simulink subsystem "PID_mask"  (R2022b)
settings: Solver=VariableStepAuto  StartTime=0.0  StopTime=10.0  RelTol=1e-3
model mask{Fd=0, F=0}
  mask prompts: Fd "Form"
settings Model: Creator=MAAM  LastModifiedBy=MAAM

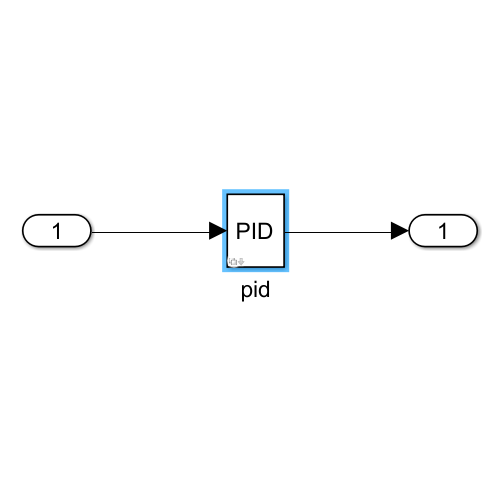
[thumbnail: Simulink's stored preview of the top-level diagram]
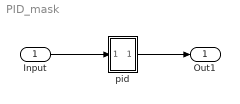
== system PID_mask ==
  Input : Inport
  pid : Subsystem  Variant=on  mask{F=Parallel, P=1, I=0, D=0}
      mask prompts: F "Form"; P "Propotional (P):"; I "Integral      (I):"; D "Drivative    (D):"
      mask init:
      | % Ensure parameters are initialized correctly
      | if isempty(P)
      |     P = 0;
      | end
      | if isempty(I)
      |     I = 0;
      | end
      | if isempty(D)
      |     D = 0;
      | end
      mask TypeOptions F: Parallel | Series | Ideal
      mask TypeOptions P: Subsystem/Gain/Gain | Subsystem1/Gain/Gain | Subsystem2/Gain/Gain
      mask TypeOptions I: Subsystem/Gain1/Gain | Subsystem1/Gain1/Gain | Subsystem2/Gain1/Gain
      mask TypeOptions D: Subsystem/Gain2/Gain | Subsystem1/Gain2/Gain | Subsystem2/Gain2/Gain
      mask Display: fprintf('PID');
  Out1 : Outport
  wires:
  pid/1(Out1) -> Out1/1
  Input/1 -> pid/1(In1)

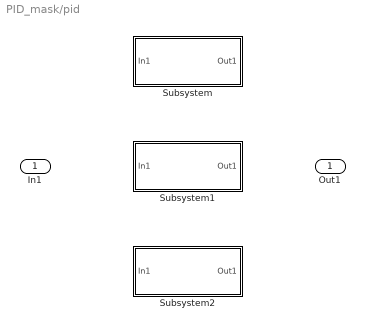
== system PID_mask/pid ==
  In1 : Inport
  Subsystem : Subsystem  VariantControl=F==1
  Subsystem1 : Subsystem  VariantControl=F==2
  Subsystem2 : Subsystem  VariantControl=F==3
  Out1 : Outport

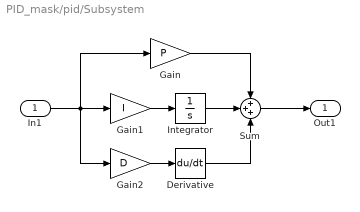
== system PID_mask/pid/Subsystem ==
  In1 : Inport
  Derivative : Derivative
  Gain : Gain  Gain=P
  Gain1 : Gain  Gain=I
  Gain2 : Gain  Gain=D
  Integrator : Integrator
  Sum : Sum  Inputs=+++
  Out1 : Outport
  wires:
  In1/1 -> Gain1/1, Gain2/1, Gain/1
  Derivative/1 -> Sum/3
  Gain/1 -> Sum/1
  Integrator/1 -> Sum/2
  Sum/1 -> Out1/1
  Gain2/1 -> Derivative/1
  Gain1/1 -> Integrator/1

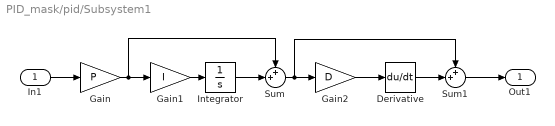
== system PID_mask/pid/Subsystem1 ==
  In1 : Inport
  Derivative : Derivative
  Gain : Gain  Gain=P
  Gain1 : Gain  Gain=I
  Gain2 : Gain  Gain=D
  Integrator : Integrator
  Sum : Sum  Inputs=++|
  Sum1 : Sum  Inputs=++|
  Out1 : Outport
  wires:
  Derivative/1 -> Sum1/2
  Sum1/1 -> Out1/1
  In1/1 -> Gain/1
  Gain1/1 -> Integrator/1
  Integrator/1 -> Sum/2
  Gain/1 -> Gain1/1, Sum/1
  Gain2/1 -> Derivative/1
  Sum/1 -> Gain2/1, Sum1/1

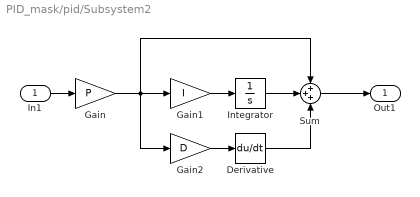
== system PID_mask/pid/Subsystem2 ==
  In1 : Inport
  Derivative : Derivative
  Gain : Gain  Gain=P
  Gain1 : Gain  Gain=I
  Gain2 : Gain  Gain=D
  Integrator : Integrator
  Sum : Sum  Inputs=+++
  Out1 : Outport
  wires:
  In1/1 -> Gain/1
  Sum/1 -> Out1/1
  Derivative/1 -> Sum/3
  Gain2/1 -> Derivative/1
  Integrator/1 -> Sum/2
  Gain1/1 -> Integrator/1
  Gain/1 -> Sum/1, Gain1/1, Gain2/1
